simulink model "Motor_Model_lag"  (Simulink 7.5)
settings: Solver=ode45  StartTime=0.0  StopTime=10.0  RelTol=1e-3
undefined symbols (not defined in the file or in its folder): b, J, K, L, R
settings Model: Creator=maen  LastModifiedBy=Rick

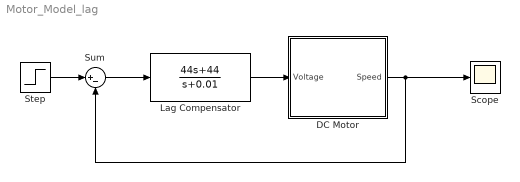
== system Motor_Model_lag ==
  DC Motor : Subsystem
  Lag Compensator : TransferFcn  Numerator=[44 44]  Denominator=[1 0.01]
  Scope : Scope
      settings: YMin=0.99945  YMax=0.99952
  Step : Step  Time=0  SampleTime=0
  Sum : Sum  Inputs=|+-  OutDataType=fixdt(1, 16)  OutScaling=2^0
  wires:
  Lag Compensator/1 -> DC Motor/1(Voltage)
  DC Motor/1(" Speed") -> Sum/2, Scope/1
  Step/1 -> Sum/1
  Sum/1 -> Lag Compensator/1

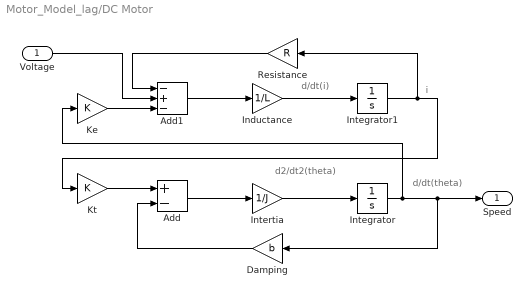
== system Motor_Model_lag/DC Motor ==
  note: i
  note: d/dt(theta)
  note: d2/dt2(theta)
  note: d/dt(i)
  Voltage : Inport  OutDataType=fixdt(1, 16)  OutScaling=2^0
  Add : Sum  Inputs=+-  OutDataType=fixdt(1, 16)  OutScaling=2^-10
  Add1 : Sum  Inputs=-+-  OutDataType=fixdt(1, 16)  OutScaling=2^-10
  Damping : Gain  Gain=b  ParameterDataType=fixdt(1, 16)  ParameterScaling=2^0  OutDataType=fixdt(1, 16)  OutScaling=2^0
  Inductance : Gain  Gain=1/L  ParameterDataType=fixdt(1, 16)  ParameterScaling=2^0  OutDataType=fixdt(1, 16)  OutScaling=2^0
  Integrator : Integrator
  Integrator1 : Integrator
  Intertia : Gain  Gain=1/J  ParameterDataType=fixdt(1, 16)  ParameterScaling=2^0  OutDataType=fixdt(1, 16)  OutScaling=2^0
  Ke : Gain  Gain=K  ParameterDataType=fixdt(1, 16)  ParameterScaling=2^0  OutDataType=fixdt(1, 16)  OutScaling=2^0
  Kt : Gain  Gain=K  ParameterDataType=fixdt(1, 16)  ParameterScaling=2^0  OutDataType=fixdt(1, 16)  OutScaling=2^0
  Resistance : Gain  Gain=R  ParameterDataType=fixdt(1, 16)  ParameterScaling=2^0  OutDataType=fixdt(1, 16)  OutScaling=2^0
  " Speed" : Outport  OutDataType=fixdt(1, 16)  OutScaling=2^0
  wires:
  Integrator1/1 -> Kt/1, Resistance/1
  Inductance/1 -> Integrator1/1
  Intertia/1 -> Integrator/1
  Integrator/1 -> Ke/1, Damping/1, " Speed"/1
  Add1/1 -> Inductance/1
  Add/1 -> Intertia/1
  Damping/1 -> Add/2
  Kt/1 -> Add/1
  Resistance/1 -> Add1/1
  Ke/1 -> Add1/3
  Voltage/1 -> Add1/2
